simulink model "MidSnap"  (R2020a)
settings: Solver=FixedStepAuto  StartTime=0.0  StopTime=10.0  FixedStep=0.1  MaxStep=0.1  RelTol=1e-3
model workspace (MAT data in the model file):
  midSnapParam = Simulink.Parameter
  midSnapParam.Value = 3
  midSnapParam.DataType = 'int32'
  midSnapParam.Dimensions = [1 1]
settings Model: DataDictionary=TestConfig.sldd  ParameterArgumentNames=midSnapParam  OrderedModelArguments=off  Creator=raarenst  LastModifiedBy=toma
settings OptimizationCC: DefaultParameterBehavior=Inlined  EnhancedBackFolding=on  PassReuseOutputArgsAs=Individual arguments  ZeroExternalMemoryAtStartup=off  ZeroInternalMemoryAtStartup=off  OptimizeBlockOrder=speed  DifferentSizesBufferReuse=on  OptimizationCustomize=off  EfficientTunableParamExpr=on
settings DebuggingCC: UnderspecifiedInitializationDetection=Classic  MergeDetectMultiDrivingBlocksExec=none  ParameterTunabilityLossMsg=error  ModelReferenceSymbolNameMessage=none
settings ModelReferenceCC: PropagateSignalLabelsOutOfModel=off
settings SFSimCC: MATLABDynamicMemAlloc=off
settings RTWCC: Description=CIGRE export target  SystemTargetFile=cigre.tlc  TemplateMakefile=cigre_tmf  Toolchain=CIGRE DLL - Microsoft Visual C++ 2019 (64bit) | nmake makefile (64-bit Windows)
settings CodeAppCC: ForceParamTrailComments=on  IgnoreCustomStorageClasses=off  OperatorAnnotations=on  SimulinkDataObjDesc=on  SFDataObjDesc=on  InsertBlockDesc=on
settings STFCustomTargetCC: TargetLangStandard=C99 (ISO)  MultiwordLength=256  GenerateSampleERTMain=on  CompOptLevelCompliant=on  CombineOutputUpdateFcns=on  ERTCustomFileBanners=on  MultiInstanceERTCode=on  CodeInterfacePackaging=Reusable function  SupportContinuousTime=off  SupportNonInlinedSFcns=off  RemoveResetFunc=on  MATLABClassNameForMDSCustomization=Simulink.SoftwareTarget.ERTCustomization  UseToolchainInfoCompliant=on  SystemTargetFile=cigre.tlc
settings ERTTargetCC: TargetLangStandard=C99 (ISO)  GenerateSampleERTMain=on  ParMdlRefBuildCompliant=off  ConcurrentExecutionCompliant=off  MultiInstanceERTCode=on  CodeInterfacePackaging=Reusable function  ModelStepFunctionPrototypeControlCompliant=off  CPPClassGenCompliant=off  InlinedParameterPlacement=NonHierarchical  RootIOFormat=Structure reference  ERTCustomFileTemplate=example_file_process.tlc

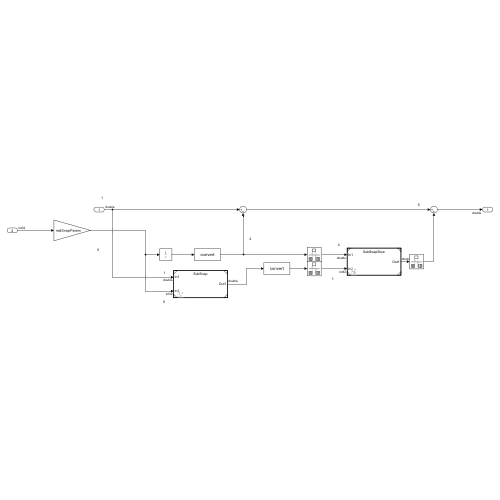
[thumbnail: Simulink's stored preview of the top-level diagram]
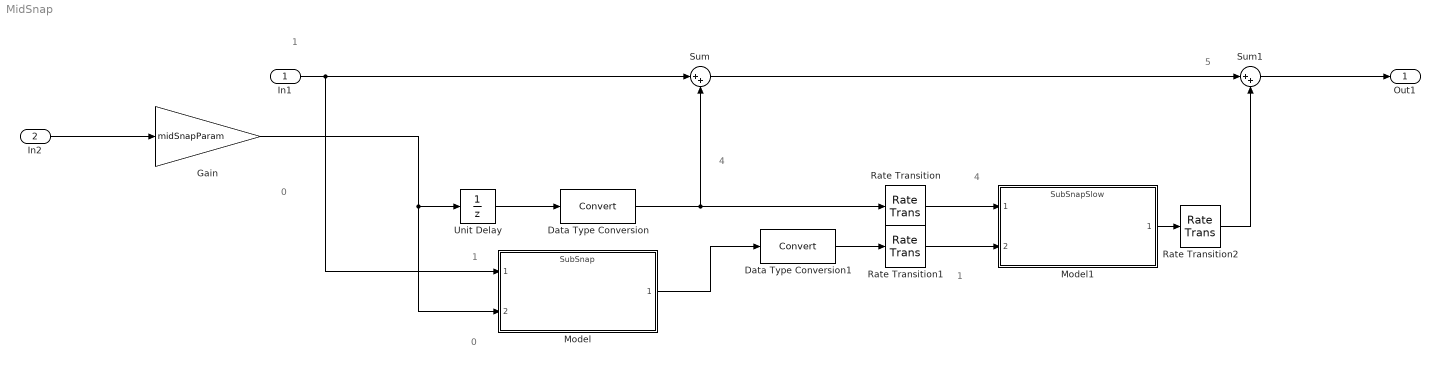
== system MidSnap ==
  note: 1
  note: 5
  note: 4
  note: 0
  note: 1
  note: 0
  note: 1
  note: 4
  In1 : Inport  OutDataTypeStr=double  SampleTime=0.1
  In2 : Inport  Port=2  OutDataTypeStr=int32  SampleTime=0.1
  Data Type Conversion : DataTypeConversion
  Data Type Conversion1 : DataTypeConversion
  Gain : Gain  Gain=midSnapParam  OutDataTypeStr=int32
  Model : ModelReference  ModelNameDialog=SubSnap  SimulationMode=Normal  ModelReferenceVersion=1.3
  Model1 : ModelReference  ModelNameDialog=SubSnapSlow  SimulationMode=Normal  ModelReferenceVersion=1.3
  Rate Transition : RateTransition
  Rate Transition1 : RateTransition
  Rate Transition2 : RateTransition
  Sum : Sum  Inputs=|++
  Sum1 : Sum  Inputs=|++
  Unit Delay : UnitDelay  InitialCondition=4  SampleTime=-1  HasFrameUpgradeWarning=on
  Out1 : Outport  OutDataTypeStr=double
  wires:
  In2/1 -> Gain/1
  Gain/1 -> Unit Delay/1, Model/2
  Unit Delay/1 -> Data Type Conversion/1
  In1/1 -> Sum/1, Model/1
  Data Type Conversion/1 -> Rate Transition/1, Sum/2
  Sum/1 -> Sum1/1
  Model/1 -> Data Type Conversion1/1
  Sum1/1 -> Out1/1
  Model1/1 -> Rate Transition2/1
  Data Type Conversion1/1 -> Rate Transition1/1
  Rate Transition/1 -> Model1/1
  Rate Transition1/1 -> Model1/2
  Rate Transition2/1 -> Sum1/2
